simulink model "sm_car"  (R2024a)
settings: Solver=ode23t  StartTime=0.0  StopTime=25  MaxStep=0.4  RelTol=1e-3  AbsTol=1e-3  EnableMultiTasking=on
PreLoadFcn:
  | % Due to usability issue in Repeating Sequence block
  | warning('off','Simulink:Masking:Invalid');
  | 
  | % Eliminate unnecessary warnings in inactive variants
  | % Warnings generated only if you click through inactive variant
  | warning('off','MATLAB:nonExistentField');
  | warning('off','Simulink:Parameters:BlkParamUndefined');
PostLoadFcn:
  | set_param([bdroot '/Vehicle'],'popup_trailer','Off')
  | warning('off','sm:sli:setup:compile:LocalSolverNotSupported')
  | %sm_car_config_maneuver(bdroot,'WOT Braking');
  | sm_car_config_vehicle(bdroot,'false');
  | sm_car_config_logging(bdroot);
InitFcn:
  | sm_car_config_camera;
  | Vehicle = sm_car_vehcfg_checkConfig(Vehicle);
  | sm_car_check_tire_model(bdroot);
StartFcn:
  | tic;
StopFcn:
  | Elapsed_Sim_Time = toc;
  | % disp(['Elapsed Sim Time = ' num2str(Elapsed_Sim_Time)]);
values from neighbouring files (symbols this model uses):
  EFFECTIVE_ROLLING_RADIUS_OF_TIRES_M = 0.23323    [vehicle_specs.m]
  TARGET_SLIP_RATIO = 0.10    (= 0.1)    [vehicle_specs.m]
undefined symbols (not defined in the file or in its folder): Axle1D, AxleIn, Camera, Control, Driver, Init, Maneuver, MAXIMUM_CONTINUOUS_CURRENT_DRAW_A, MAXIMUM_NEGATIVE_TORQUE_FROM_MOTOR_Nm, MAXIMUM_TORQUE_FROM_MOTOR_Nm, Pedal, RaceFix, RaceSpin, Scene, ShaftL1, ShaftL2, ShaftR1, ShaftR2, Visual, X, xy_data_car_side, Y, Z
libraries: sm_lib x1112, nesl_utility x285, fl_lib x221, simulink x24, sdl_lib x16, SimscapeFluids_lib x9, ee_lib x5, Linkage_Systems x4, Tire_1x2x x4, simulink_extras x3, slpidlib x2, AntiRollBar_Systems x2
(part 9 of 43)

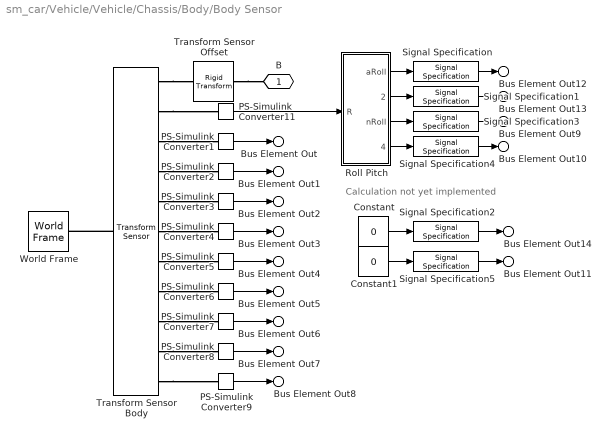
== system sm_car/Vehicle/Vehicle/Chassis/Body/Body Sensor ==
  note: Calculation not yet implemented
  Constant : Constant  Value=0
  Constant1 : Constant  Value=0
  PS-Simulink Converter1 : nesl_utility/PS-Simulink Converter  PhysicalDomain=network_engine_domain  SubClassName=ps_output  LeftPortType=input  RightPortType=output  PseudoPeriodic=off  Frequencies=[]  VectorFormat=1-D array  Unit=m  AffineConversion=off
  PS-Simulink Converter11 : nesl_utility/PS-Simulink Converter  PhysicalDomain=network_engine_domain  SubClassName=ps_output  LeftPortType=input  RightPortType=output  PseudoPeriodic=off  Frequencies=[]  VectorFormat=1-D array  Unit=1  AffineConversion=off
  PS-Simulink Converter2 : nesl_utility/PS-Simulink Converter  PhysicalDomain=network_engine_domain  SubClassName=ps_output  LeftPortType=input  RightPortType=output  PseudoPeriodic=off  Frequencies=[]  VectorFormat=1-D array  Unit=m  AffineConversion=off
  PS-Simulink Converter3 : nesl_utility/PS-Simulink Converter  PhysicalDomain=network_engine_domain  SubClassName=ps_output  LeftPortType=input  RightPortType=output  PseudoPeriodic=off  Frequencies=[]  VectorFormat=1-D array  Unit=m  AffineConversion=off
  PS-Simulink Converter4 : nesl_utility/PS-Simulink Converter  PhysicalDomain=network_engine_domain  SubClassName=ps_output  LeftPortType=input  RightPortType=output  PseudoPeriodic=off  Frequencies=[]  VectorFormat=1-D array  Unit=m/s  AffineConversion=off
  PS-Simulink Converter5 : nesl_utility/PS-Simulink Converter  PhysicalDomain=network_engine_domain  SubClassName=ps_output  LeftPortType=input  RightPortType=output  PseudoPeriodic=off  Frequencies=[]  VectorFormat=1-D array  Unit=m/s  AffineConversion=off
  PS-Simulink Converter6 : nesl_utility/PS-Simulink Converter  PhysicalDomain=network_engine_domain  SubClassName=ps_output  LeftPortType=input  RightPortType=output  PseudoPeriodic=off  Frequencies=[]  VectorFormat=1-D array  Unit=m/s  AffineConversion=off
  PS-Simulink Converter7 : nesl_utility/PS-Simulink Converter  PhysicalDomain=network_engine_domain  SubClassName=ps_output  LeftPortType=input  RightPortType=output  PseudoPeriodic=off  Frequencies=[]  VectorFormat=1-D array  Unit=m/s^2  AffineConversion=off
  PS-Simulink Converter8 : nesl_utility/PS-Simulink Converter  PhysicalDomain=network_engine_domain  SubClassName=ps_output  LeftPortType=input  RightPortType=output  PseudoPeriodic=off  Frequencies=[]  VectorFormat=1-D array  Unit=m/s^2  AffineConversion=off
  PS-Simulink Converter9 : nesl_utility/PS-Simulink Converter  PhysicalDomain=network_engine_domain  SubClassName=ps_output  LeftPortType=input  RightPortType=output  PseudoPeriodic=off  Frequencies=[]  VectorFormat=1-D array  Unit=m/s^2  AffineConversion=off
  Roll Pitch : Subsystem
  Signal Specification : SignalSpecification  Unit=rad
  Signal Specification1 : SignalSpecification  Unit=rad
  Signal Specification2 : SignalSpecification  Unit=rad
  Signal Specification3 : SignalSpecification  Unit=rad/s
  Signal Specification4 : SignalSpecification  Unit=rad/s
  Signal Specification5 : SignalSpecification  Unit=rad/s
  Transform Sensor Offset : sm_lib/Frames and Transforms/Rigid Transform  RotationMethod=None  FollAlignAxisA=+X  BaseAlignAxisA=+Y  FollAlignAxisB=+Y  BaseAlignAxisB=+Z  RotationStandardAxis=+Z  RotationAngle=0.0  RotationAngleUnits=deg  RotationArbitraryAxis=[0 0 1]  RotationSequenceAxes=FollowerAxes  RotationSequence=XYX  RotationSequenceAngles=[0 0 0]  RotationSequenceAnglesUnits=deg  RotationMatrix=[1 0 0; 0 1 0; 0 0 1]  Quaternion=[1 0 0 0]  TranslationMethod=Cartesian  TranslationCartesianOffset=offset_body_sensor  TranslationCartesianOffsetUnits=m  TranslationStandardAxis=+Z  TranslationStandardOffset=0  TranslationStandardOffsetUnits=m  TranslationROffset=0  TranslationROffsetUnits=m  TranslationThetaOffset=0  TranslationThetaOffsetUnits=deg  TranslationZOffset=0  TranslationZOffsetUnits=m
  Transform Sensor Body : sm_lib/Frames and Transforms/Transform Sensor  MeasurementFrame=NonRotatingFollower  RotationSequence=XYX  SenseAngle=off  SenseAxis=off  SenseQ=off  SenseR=on  SenseRotationSequence=off  SenseOmegaX=off  SenseOmegaY=off  SenseOmegaZ=off  SenseOmega=off  SenseQDot=off  SenseRDot=off  SenseRotationSequenceDot=off  SenseAlphaX=off  SenseAlphaY=off  SenseAlphaZ=off  SenseAlpha=off  SenseQDDot=off  SenseRDDot=off  SenseX=on  SenseY=on  SenseZ=on  SenseXYZ=off  SenseRad=off  SenseAzim=off  SenseDist=off  SenseInc=off  SenseXDot=on  SenseYDot=on  SenseZDot=on  SenseXYZDot=off  SenseRadDot=off  SenseAzimDot=off  SenseDistDot=off  SenseIncDot=off  SenseXDDot=on  SenseYDDot=on  SenseZDDot=on  SenseXYZDDot=off  SenseRadDDot=off  SenseAzimDDot=off  SenseDistDDot=off  SenseIncDDot=off
  World Frame : sm_lib/Frames and Transforms/World Frame
  B : PMIOPort  Side=Left
  Bus Element Out : Outport  VectorParamsAs1DForOutWhenUnconnected=off  PortName=Body  Element=x
  Bus Element Out1 : Outport  VectorParamsAs1DForOutWhenUnconnected=off  PortName=Body  Element=y
  Bus Element Out2 : Outport  VectorParamsAs1DForOutWhenUnconnected=off  PortName=Body  Element=z
  Bus Element Out3 : Outport  VectorParamsAs1DForOutWhenUnconnected=off  PortName=Body  Element=vx
  Bus Element Out4 : Outport  VectorParamsAs1DForOutWhenUnconnected=off  PortName=Body  Element=vy
  Bus Element Out5 : Outport  VectorParamsAs1DForOutWhenUnconnected=off  PortName=Body  Element=vz
  Bus Element Out6 : Outport  VectorParamsAs1DForOutWhenUnconnected=off  PortName=Body  Element=gx
  Bus Element Out7 : Outport  VectorParamsAs1DForOutWhenUnconnected=off  PortName=Body  Element=gy
  Bus Element Out8 : Outport  VectorParamsAs1DForOutWhenUnconnected=off  PortName=Body  Element=gz
  Bus Element Out9 : Outport  VectorParamsAs1DForOutWhenUnconnected=off  PortName=Body  Element=nRoll
  Bus Element Out10 : Outport  VectorParamsAs1DForOutWhenUnconnected=off  PortName=Body  Element=nPitch
  Bus Element Out11 : Outport  VectorParamsAs1DForOutWhenUnconnected=off  PortName=Body  Element=nYaw
  Bus Element Out12 : Outport  VectorParamsAs1DForOutWhenUnconnected=off  PortName=Body  Element=aRoll
  Bus Element Out13 : Outport  VectorParamsAs1DForOutWhenUnconnected=off  PortName=Body  Element=aPitch
  Bus Element Out14 : Outport  VectorParamsAs1DForOutWhenUnconnected=off  PortName=Body  Element=aYaw
  wires:
  PS-Simulink Converter9/1 -> Bus Element Out8/1
  PS-Simulink Converter11/1 -> Roll Pitch/1(R)
  PS-Simulink Converter6/1 -> Bus Element Out5/1
  PS-Simulink Converter7/1 -> Bus Element Out6/1
  PS-Simulink Converter2/1 -> Bus Element Out1/1
  PS-Simulink Converter8/1 -> Bus Element Out7/1
  PS-Simulink Converter5/1 -> Bus Element Out4/1
  PS-Simulink Converter3/1 -> Bus Element Out2/1
  PS-Simulink Converter1/1 -> Bus Element Out/1
  PS-Simulink Converter4/1 -> Bus Element Out3/1
  Signal Specification/1 -> Bus Element Out12/1
  Signal Specification1/1 -> Bus Element Out13/1
  Signal Specification2/1 -> Bus Element Out14/1
  Signal Specification3/1 -> Bus Element Out9/1
  Signal Specification4/1 -> Bus Element Out10/1
  Signal Specification5/1 -> Bus Element Out11/1
  Constant/1 -> Signal Specification2/1
  Constant1/1 -> Signal Specification5/1
  Roll Pitch/3(nRoll) -> Signal Specification3/1
  Roll Pitch/4(nPitch) -> Signal Specification4/1
  Roll Pitch/2(aPitch) -> Signal Specification1/1
  Roll Pitch/1(aRoll) -> Signal Specification/1
  connections:
  Transform Sensor Body/RConn5 -- PS-Simulink Converter3/LConn1
  Transform Sensor Body/RConn4 -- PS-Simulink Converter2/LConn1
  Transform Sensor Body/RConn11 -- PS-Simulink Converter9/LConn1
  Transform Sensor Body/RConn2 -- PS-Simulink Converter11/LConn1
  Transform Sensor Body/RConn7 -- PS-Simulink Converter5/LConn1
  Transform Sensor Body/RConn3 -- PS-Simulink Converter1/LConn1
  Transform Sensor Body/LConn1 -- World Frame/RConn1
  Transform Sensor Offset/LConn1 -- B/RConn1
  Transform Sensor Body/RConn10 -- PS-Simulink Converter8/LConn1
  Transform Sensor Body/RConn9 -- PS-Simulink Converter7/LConn1
  Transform Sensor Body/RConn8 -- PS-Simulink Converter6/LConn1
  Transform Sensor Body/RConn6 -- PS-Simulink Converter4/LConn1
  Transform Sensor Body/RConn1 -- Transform Sensor Offset/RConn1

== system sm_car/Vehicle/Vehicle/Chassis/Body/Passenger FL ==
  None : Subsystem  VariantControl=None
      mask Display: disp(' ')
  P : PMIOPort  Side=Left
  m : Outport  VectorParamsAs1DForOutWhenUnconnected=off

== system sm_car/Vehicle/Vehicle/Chassis/Body/Passenger FR ==
  None : Subsystem  VariantControl=None
      mask Display: disp(' ')
  P : PMIOPort  Side=Left
  m : Outport  VectorParamsAs1DForOutWhenUnconnected=off

== system sm_car/Vehicle/Vehicle/Chassis/Body/Passenger RL ==
  None : Subsystem  VariantControl=None
      mask Display: disp(' ')
  P : PMIOPort  Side=Left
  m : Outport  VectorParamsAs1DForOutWhenUnconnected=off

== system sm_car/Vehicle/Vehicle/Chassis/Body/Passenger RR ==
  None : Subsystem  VariantControl=None
      mask Display: disp(' ')
  P : PMIOPort  Side=Left
  m : Outport  VectorParamsAs1DForOutWhenUnconnected=off

== system sm_car/Vehicle/Vehicle/Chassis/Damper/Decoupled ==
  In Bus Element1 : Inport  PortName=Ctrl  Element=L1
  In Bus Element : Inport  PortName=Ctrl  Element=R1
  In Bus Element2 : Inport  PortName=Ctrl  Element=L2
  In Bus Element3 : Inport  PortName=Ctrl  Element=R2
  Damper A1 Heave : Subsystem  Variant=on  VariantControlMode=label  VariantControl=Variant1  LabelModeActiveChoice=Linear  mask(Variants for Damper){Damper=Damper.Axle1.Heave, VariantLabel=Damper.Axle1.Heave.class.Value}
      mask prompts: Damper "Damper Parameters"; VariantLabel "Variant Label"
      mask help: Select option and provide parameters for damper. Option is chosen by string provided in Variant Label. The parameters for the selected option is contained in Damper data structure.
      mask init:
      | curblk = gcb;
      | 
      | % Set variant for this block 
      | set_param(curblk,'LabelModeActiveChoice',VariantLabel);
      settings: AttributesFormatString=%<ActiveVariant>
      mask Display: disp(' ')
  Damper A1 Roll : Subsystem  Variant=on  VariantControlMode=label  VariantControl=Variant1  LabelModeActiveChoice=Linear  mask(Variants for Damper){Damper=Damper.Axle1.Roll, VariantLabel=Damper.Axle1.Roll.class.Value}
      mask prompts: Damper "Damper Parameters"; VariantLabel "Variant Label"
      mask help: Select option and provide parameters for damper. Option is chosen by string provided in Variant Label. The parameters for the selected option is contained in Damper data structure.
      mask init:
      | curblk = gcb;
      | 
      | % Set variant for this block 
      | set_param(curblk,'LabelModeActiveChoice',VariantLabel);
      settings: AttributesFormatString=%<ActiveVariant>
      mask Display: disp(' ')
  Damper A2 Heave : Subsystem  Variant=on  VariantControlMode=label  VariantControl=Variant1  LabelModeActiveChoice=Linear  mask(Variants for Damper){Damper=Damper.Axle2.Heave, VariantLabel=Damper.Axle2.Heave.class.Value}
      mask prompts: Damper "Damper Parameters"; VariantLabel "Variant Label"
      mask help: Select option and provide parameters for damper. Option is chosen by string provided in Variant Label. The parameters for the selected option is contained in Damper data structure.
      mask init:
      | curblk = gcb;
      | 
      | % Set variant for this block 
      | set_param(curblk,'LabelModeActiveChoice',VariantLabel);
      settings: AttributesFormatString=%<ActiveVariant>
      mask Display: disp(' ')
  Damper A2 Roll : Subsystem  Variant=on  VariantControlMode=label  VariantControl=Variant1  LabelModeActiveChoice=Linear  mask(Variants for Damper){Damper=Damper.Axle2.Roll, VariantLabel=Damper.Axle2.Roll.class.Value}
      mask prompts: Damper "Damper Parameters"; VariantLabel "Variant Label"
      mask help: Select option and provide parameters for damper. Option is chosen by string provided in Variant Label. The parameters for the selected option is contained in Damper data structure.
      mask init:
      | curblk = gcb;
      | 
      | % Set variant for this block 
      | set_param(curblk,'LabelModeActiveChoice',VariantLabel);
      settings: AttributesFormatString=%<ActiveVariant>
      mask Display: disp(' ')
  MTRef L1 : fl_lib/Mechanical/Translational Elements/Mechanical Translational Reference
  MTRef L2 : fl_lib/Mechanical/Translational Elements/Mechanical Translational Reference
  MTRef R1 : fl_lib/Mechanical/Translational Elements/Mechanical Translational Reference
  MTRef R2 : fl_lib/Mechanical/Translational Elements/Mechanical Translational Reference
  L1 : PMIOPort  Side=Left
  R1 : PMIOPort  Port=2  Side=Right
  L2 : PMIOPort  Port=3  Side=Left
  R2 : PMIOPort  Port=4  Side=Right
  Out Bus Element : Outport  VectorParamsAs1DForOutWhenUnconnected=off  PortName=meas  Element=L1
  Out Bus Element1 : Outport  VectorParamsAs1DForOutWhenUnconnected=off  PortName=meas  Element=R1
  Out Bus Element2 : Outport  VectorParamsAs1DForOutWhenUnconnected=off  PortName=meas  Element=L2
  Out Bus Element3 : Outport  VectorParamsAs1DForOutWhenUnconnected=off  PortName=meas  Element=R2
  wires:
  In Bus Element/1 -> Damper A1 Roll/1("Ctrl ")
  In Bus Element1/1 -> Damper A1 Heave/1("Ctrl ")
  Damper A1 Heave/1(" meas") -> Out Bus Element/1
  Damper A1 Roll/1(" meas") -> Out Bus Element1/1
  In Bus Element3/1 -> Damper A2 Roll/1("Ctrl ")
  In Bus Element2/1 -> Damper A2 Heave/1("Ctrl ")
  Damper A2 Heave/1(" meas") -> Out Bus Element2/1
  Damper A2 Roll/1(" meas") -> Out Bus Element3/1
  connections:
  Damper A1 Roll/LConn1 -- R1/RConn1
  Damper A1 Roll/RConn1 -- MTRef R1/LConn1
  Damper A2 Roll/LConn1 -- R2/RConn1
  Damper A2 Roll/RConn1 -- MTRef R2/LConn1
  Damper A2 Heave/LConn1 -- L2/RConn1
  Damper A2 Heave/RConn1 -- MTRef L2/LConn1
  Damper A1 Heave/LConn1 -- L1/RConn1
  Damper A1 Heave/RConn1 -- MTRef L1/LConn1

== system sm_car/Vehicle/Vehicle/Chassis/Damper/Independent ==
  In Bus Element1 : Inport  PortName=Ctrl  Element=L1
  In Bus Element : Inport  PortName=Ctrl  Element=R1
  In Bus Element2 : Inport  PortName=Ctrl  Element=L2
  In Bus Element3 : Inport  PortName=Ctrl  Element=R2
  Damper L1 : Subsystem  Variant=on  VariantControlMode=label  VariantControl=Variant1  LabelModeActiveChoice=Linear  mask(Variants for Damper){Damper=Damper.Axle1, VariantLabel=Damper.Axle1.class.Value}
      mask prompts: Damper "Damper Parameters"; VariantLabel "Variant Label"
      mask help: Select option and provide parameters for damper. Option is chosen by string provided in Variant Label. The parameters for the selected option is contained in Damper data structure.
      mask init:
      | curblk = gcb;
      | 
      | % Set variant for this block 
      | set_param(curblk,'LabelModeActiveChoice',VariantLabel);
      settings: AttributesFormatString=%<ActiveVariant>
      mask Display: disp(' ')
  Damper L2 : Subsystem  Variant=on  VariantControlMode=label  VariantControl=Variant1  LabelModeActiveChoice=Linear  mask(Variants for Damper){Damper=Damper.Axle2, VariantLabel=Damper.Axle2.class.Value}
      mask prompts: Damper "Damper Parameters"; VariantLabel "Variant Label"
      mask help: Select option and provide parameters for damper. Option is chosen by string provided in Variant Label. The parameters for the selected option is contained in Damper data structure.
      mask init:
      | curblk = gcb;
      | 
      | % Set variant for this block 
      | set_param(curblk,'LabelModeActiveChoice',VariantLabel);
      settings: AttributesFormatString=%<ActiveVariant>
      mask Display: disp(' ')
  Damper R1 : Subsystem  Variant=on  VariantControlMode=label  VariantControl=Variant1  LabelModeActiveChoice=Linear  mask(Variants for Damper){Damper=Damper.Axle1, VariantLabel=Damper.Axle1.class.Value}
      mask prompts: Damper "Damper Parameters"; VariantLabel "Variant Label"
      mask help: Select option and provide parameters for damper. Option is chosen by string provided in Variant Label. The parameters for the selected option is contained in Damper data structure.
      mask init:
      | curblk = gcb;
      | 
      | % Set variant for this block 
      | set_param(curblk,'LabelModeActiveChoice',VariantLabel);
      settings: AttributesFormatString=%<ActiveVariant>
      mask Display: disp(' ')
  Damper R2 : Subsystem  Variant=on  VariantControlMode=label  VariantControl=Variant1  LabelModeActiveChoice=Linear  mask(Variants for Damper){Damper=Damper.Axle2, VariantLabel=Damper.Axle2.class.Value}
      mask prompts: Damper "Damper Parameters"; VariantLabel "Variant Label"
      mask help: Select option and provide parameters for damper. Option is chosen by string provided in Variant Label. The parameters for the selected option is contained in Damper data structure.
      mask init:
      | curblk = gcb;
      | 
      | % Set variant for this block 
      | set_param(curblk,'LabelModeActiveChoice',VariantLabel);
      settings: AttributesFormatString=%<ActiveVariant>
      mask Display: disp(' ')
  MTRef L1 : fl_lib/Mechanical/Translational Elements/Mechanical Translational Reference
  MTRef L2 : fl_lib/Mechanical/Translational Elements/Mechanical Translational Reference
  MTRef R1 : fl_lib/Mechanical/Translational Elements/Mechanical Translational Reference
  MTRef R2 : fl_lib/Mechanical/Translational Elements/Mechanical Translational Reference
  L1 : PMIOPort  Side=Left
  R1 : PMIOPort  Port=2  Side=Right
  L2 : PMIOPort  Port=3  Side=Left
  R2 : PMIOPort  Port=4  Side=Right
  Out Bus Element : Outport  VectorParamsAs1DForOutWhenUnconnected=off  PortName=meas  Element=L1
  Out Bus Element1 : Outport  VectorParamsAs1DForOutWhenUnconnected=off  PortName=meas  Element=R1
  Out Bus Element2 : Outport  VectorParamsAs1DForOutWhenUnconnected=off  PortName=meas  Element=L2
  Out Bus Element3 : Outport  VectorParamsAs1DForOutWhenUnconnected=off  PortName=meas  Element=R2
  wires:
  In Bus Element/1 -> Damper R1/1("Ctrl ")
  In Bus Element1/1 -> Damper L1/1("Ctrl ")
  Damper L1/1(" meas") -> Out Bus Element/1
  Damper R1/1(" meas") -> Out Bus Element1/1
  In Bus Element3/1 -> Damper R2/1("Ctrl ")
  In Bus Element2/1 -> Damper L2/1("Ctrl ")
  Damper L2/1(" meas") -> Out Bus Element2/1
  Damper R2/1(" meas") -> Out Bus Element3/1
  connections:
  Damper R1/LConn1 -- R1/RConn1
  Damper R1/RConn1 -- MTRef R1/LConn1
  Damper R2/LConn1 -- R2/RConn1
  Damper R2/RConn1 -- MTRef R2/LConn1
  Damper L2/LConn1 -- L2/RConn1
  Damper L2/RConn1 -- MTRef L2/LConn1
  Damper L1/LConn1 -- L1/RConn1
  Damper L1/RConn1 -- MTRef L1/LConn1

== system sm_car/Vehicle/Vehicle/Chassis/Spring/Decoupled ==
  In Bus Element1 : Inport  PortName=Ctrl  Element=L1
  In Bus Element2 : Inport  PortName=Ctrl  Element=R1
  In Bus Element3 : Inport  PortName=Ctrl  Element=L2
  In Bus Element4 : Inport  PortName=Ctrl  Element=R2
  MTRef Heave A1 : fl_lib/Mechanical/Translational Elements/Mechanical Translational Reference
  MTRef Heave A2 : fl_lib/Mechanical/Translational Elements/Mechanical Translational Reference
  MTRef Roll A1 : fl_lib/Mechanical/Translational Elements/Mechanical Translational Reference
  MTRef Roll A2 : fl_lib/Mechanical/Translational Elements/Mechanical Translational Reference
  Spring A1 Heave : Subsystem  Variant=on  VariantControlMode=label  VariantControl=Variant1  LabelModeActiveChoice=Linear  mask(Variants for Spring){Spring=Spring.Axle1.Heave, VariantLabel=Spring.Axle1.Heave.class.Value}
      mask prompts: Spring "Spring Parameters"; VariantLabel "Variant Label"
      mask help: Select option and provide parameters for spring. Option is chosen by string provided in Variant Label. The parameters for the selected option is contained in Spring data structure.
      mask init:
      | curblk = gcb;
      | 
      | % Set variant for this block 
      | set_param(curblk,'LabelModeActiveChoice',VariantLabel);
      settings: AttributesFormatString=%<ActiveVariant>
      mask Display: disp(' ')
  Spring A1 Roll : Subsystem  Variant=on  VariantControlMode=label  VariantControl=Variant1  LabelModeActiveChoice=Linear  mask(Variants for Spring){Spring=Spring.Axle1.Roll, VariantLabel=Spring.Axle1.Roll.class.Value}
      mask prompts: Spring "Spring Parameters"; VariantLabel "Variant Label"
      mask help: Select option and provide parameters for spring. Option is chosen by string provided in Variant Label. The parameters for the selected option is contained in Spring data structure.
      mask init:
      | curblk = gcb;
      | 
      | % Set variant for this block 
      | set_param(curblk,'LabelModeActiveChoice',VariantLabel);
      settings: AttributesFormatString=%<ActiveVariant>
      mask Display: disp(' ')
  Spring A2 Heave : Subsystem  Variant=on  VariantControlMode=label  VariantControl=Variant1  LabelModeActiveChoice=Linear  mask(Variants for Spring){Spring=Spring.Axle2.Heave, VariantLabel=Spring.Axle2.Heave.class.Value}
      mask prompts: Spring "Spring Parameters"; VariantLabel "Variant Label"
      mask help: Select option and provide parameters for spring. Option is chosen by string provided in Variant Label. The parameters for the selected option is contained in Spring data structure.
      mask init:
      | curblk = gcb;
      | 
      | % Set variant for this block 
      | set_param(curblk,'LabelModeActiveChoice',VariantLabel);
      settings: AttributesFormatString=%<ActiveVariant>
      mask Display: disp(' ')
  Spring A2 Roll : Subsystem  Variant=on  VariantControlMode=label  VariantControl=Variant1  LabelModeActiveChoice=Linear  mask(Variants for Spring){Spring=Spring.Axle2.Roll, VariantLabel=Spring.Axle2.Roll.class.Value}
      mask prompts: Spring "Spring Parameters"; VariantLabel "Variant Label"
      mask help: Select option and provide parameters for spring. Option is chosen by string provided in Variant Label. The parameters for the selected option is contained in Spring data structure.
      mask init:
      | curblk = gcb;
      | 
      | % Set variant for this block 
      | set_param(curblk,'LabelModeActiveChoice',VariantLabel);
      settings: AttributesFormatString=%<ActiveVariant>
      mask Display: disp(' ')
  L1 : PMIOPort  Side=Left
  R1 : PMIOPort  Port=2  Side=Right
  L2 : PMIOPort  Port=3  Side=Left
  R2 : PMIOPort  Port=4  Side=Right
  Out Bus Element : Outport  VectorParamsAs1DForOutWhenUnconnected=off  PortName=meas  Element=L1
  Out Bus Element1 : Outport  VectorParamsAs1DForOutWhenUnconnected=off  PortName=meas  Element=R1
  Out Bus Element2 : Outport  VectorParamsAs1DForOutWhenUnconnected=off  PortName=meas  Element=L2
  Out Bus Element3 : Outport  VectorParamsAs1DForOutWhenUnconnected=off  PortName=meas  Element=R2
  wires:
  In Bus Element1/1 -> Spring A1 Heave/1("Ctrl ")
  Spring A1 Heave/1(" meas") -> Out Bus Element/1
  In Bus Element2/1 -> Spring A1 Roll/1("Ctrl ")
  Spring A1 Roll/1(" meas") -> Out Bus Element1/1
  In Bus Element3/1 -> Spring A2 Heave/1("Ctrl ")
  Spring A2 Heave/1(" meas") -> Out Bus Element2/1
  In Bus Element4/1 -> Spring A2 Roll/1("Ctrl ")
  Spring A2 Roll/1(" meas") -> Out Bus Element3/1
  connections:
  Spring A1 Roll/LConn1 -- R1/RConn1
  Spring A1 Roll/RConn1 -- MTRef Roll A1/LConn1
  Spring A2 Roll/LConn1 -- R2/RConn1
  Spring A2 Roll/RConn1 -- MTRef Roll A2/LConn1
  Spring A2 Heave/LConn1 -- L2/RConn1
  Spring A2 Heave/RConn1 -- MTRef Heave A2/LConn1
  Spring A1 Heave/LConn1 -- L1/RConn1
  Spring A1 Heave/RConn1 -- MTRef Heave A1/LConn1

== system sm_car/Vehicle/Vehicle/Chassis/Spring/Independent ==
  In Bus Element1 : Inport  PortName=Ctrl  Element=L1
  In Bus Element2 : Inport  PortName=Ctrl  Element=R1
  In Bus Element3 : Inport  PortName=Ctrl  Element=L2
  In Bus Element4 : Inport  PortName=Ctrl  Element=R2
  MTRef L1 : fl_lib/Mechanical/Translational Elements/Mechanical Translational Reference
  MTRef L2 : fl_lib/Mechanical/Translational Elements/Mechanical Translational Reference
  MTRef R1 : fl_lib/Mechanical/Translational Elements/Mechanical Translational Reference
  MTRef R2 : fl_lib/Mechanical/Translational Elements/Mechanical Translational Reference
  Spring L1 : Subsystem  Variant=on  VariantControlMode=label  VariantControl=Variant1  LabelModeActiveChoice=Linear  mask(Variants for Spring){Spring=Spring.Axle1, VariantLabel=Spring.Axle1.class.Value}
      mask prompts: Spring "Spring Parameters"; VariantLabel "Variant Label"
      mask help: Select option and provide parameters for spring. Option is chosen by string provided in Variant Label. The parameters for the selected option is contained in Spring data structure.
      mask init:
      | curblk = gcb;
      | 
      | % Set variant for this block 
      | set_param(curblk,'LabelModeActiveChoice',VariantLabel);
      settings: AttributesFormatString=%<ActiveVariant>
      mask Display: disp(' ')
  Spring L2 : Subsystem  Variant=on  VariantControlMode=label  VariantControl=Variant1  LabelModeActiveChoice=Linear  mask(Variants for Spring){Spring=Spring.Axle2, VariantLabel=Spring.Axle2.class.Value}
      mask prompts: Spring "Spring Parameters"; VariantLabel "Variant Label"
      mask help: Select option and provide parameters for spring. Option is chosen by string provided in Variant Label. The parameters for the selected option is contained in Spring data structure.
      mask init:
      | curblk = gcb;
      | 
      | % Set variant for this block 
      | set_param(curblk,'LabelModeActiveChoice',VariantLabel);
      settings: AttributesFormatString=%<ActiveVariant>
      mask Display: disp(' ')
  Spring R1 : Subsystem  Variant=on  VariantControlMode=label  VariantControl=Variant1  LabelModeActiveChoice=Linear  mask(Variants for Spring){Spring=Spring.Axle1, VariantLabel=Spring.Axle1.class.Value}
      mask prompts: Spring "Spring Parameters"; VariantLabel "Variant Label"
      mask help: Select option and provide parameters for spring. Option is chosen by string provided in Variant Label. The parameters for the selected option is contained in Spring data structure.
      mask init:
      | curblk = gcb;
      | 
      | % Set variant for this block 
      | set_param(curblk,'LabelModeActiveChoice',VariantLabel);
      settings: AttributesFormatString=%<ActiveVariant>
      mask Display: disp(' ')
  Spring R2 : Subsystem  Variant=on  VariantControlMode=label  VariantControl=Variant1  LabelModeActiveChoice=Linear  mask(Variants for Spring){Spring=Spring.Axle2, VariantLabel=Spring.Axle2.class.Value}
      mask prompts: Spring "Spring Parameters"; VariantLabel "Variant Label"
      mask help: Select option and provide parameters for spring. Option is chosen by string provided in Variant Label. The parameters for the selected option is contained in Spring data structure.
      mask init:
      | curblk = gcb;
      | 
      | % Set variant for this block 
      | set_param(curblk,'LabelModeActiveChoice',VariantLabel);
      settings: AttributesFormatString=%<ActiveVariant>
      mask Display: disp(' ')
  L1 : PMIOPort  Side=Left
  R1 : PMIOPort  Port=2  Side=Right
  L2 : PMIOPort  Port=3  Side=Left
  R2 : PMIOPort  Port=4  Side=Right
  Out Bus Element : Outport  VectorParamsAs1DForOutWhenUnconnected=off  PortName=meas  Element=L1
  Out Bus Element1 : Outport  VectorParamsAs1DForOutWhenUnconnected=off  PortName=meas  Element=R1
  Out Bus Element2 : Outport  VectorParamsAs1DForOutWhenUnconnected=off  PortName=meas  Element=L2
  Out Bus Element3 : Outport  VectorParamsAs1DForOutWhenUnconnected=off  PortName=meas  Element=R2
  wires:
  In Bus Element1/1 -> Spring L1/1("Ctrl ")
  Spring L1/1(" meas") -> Out Bus Element/1
  In Bus Element2/1 -> Spring R1/1("Ctrl ")
  Spring R1/1(" meas") -> Out Bus Element1/1
  In Bus Element3/1 -> Spring L2/1("Ctrl ")
  Spring L2/1(" meas") -> Out Bus Element2/1
  In Bus Element4/1 -> Spring R2/1("Ctrl ")
  Spring R2/1(" meas") -> Out Bus Element3/1
  connections:
  Spring R1/LConn1 -- R1/RConn1
  Spring R1/RConn1 -- MTRef R1/LConn1
  Spring R2/LConn1 -- R2/RConn1
  Spring R2/RConn1 -- MTRef R2/LConn1
  Spring L2/LConn1 -- L2/RConn1
  Spring L2/RConn1 -- MTRef L2/LConn1
  Spring L1/LConn1 -- L1/RConn1
  Spring L1/RConn1 -- MTRef L1/LConn1

== system sm_car/Vehicle/Vehicle/Chassis/SuspA1/Linkage ==
  In Bus Element : Inport  PortName=CtrlBus  Element=Steer
  DrvBus : Inport  Port=2
  Anti Roll Bar : AntiRollBar_Systems/Anti Roll Bar  LabelModeActiveChoice=Droplink  AntiRollBar=Susp.AntiRollBar  VariantLabel=Susp.AntiRollBar.class.Value
      settings: AttributesFormatString=%<LabelModeActiveChoice>
  Linkage L : Linkage_Systems/Linkage  VariantControl=Variant1  LabelModeActiveChoice=DoubleWishbone  popup_leftRight=Left  Linkage=Susp.Linkage  InitLinkage=Init  VariantLabel=Susp.Linkage.class.Value
      settings: AttributesFormatString=%<ActiveVariant>
  Linkage R : Linkage_Systems/Linkage  Tag=PublishSubsystem  VariantControl=Variant1  LabelModeActiveChoice=DoubleWishbone  popup_leftRight=Right  Linkage=Susp.Linkage  InitLinkage=Init  VariantLabel=Susp.Linkage.class.Value
      settings: AttributesFormatString=%<ActiveVariant>
  Simscape Bus L : SimscapeBus  HierarchyStrings=RaceSpin;RaceFix;Axle1D;AxleIn
  Simscape Bus L1 : SimscapeBus  HierarchyStrings=RaceSpin;RaceFix;Axle1D;AxleIn
  Steer : Subsystem  Variant=on  VariantControlMode=label  VariantControl=Steer  LabelModeActiveChoice=WheelDrivenRack1UJoint  mask{Steer=Susp.Steer, VariantLabel=Susp.Steer.class.Value}
      mask prompts: Steer "Steer Parameters"; VariantLabel "Variant Label"
      mask init:
      | curblk = gcb;
      | 
      | % Set variant for this block 
      | set_param(curblk,'LabelModeActiveChoice',VariantLabel);
      settings: AttributesFormatString=%<ActiveVariant>
      mask Display: disp(' ');
  Wheel Meas Left : Subsystem  mask(Wheel Measurements){popup_leftRight=Left}
      mask prompts: popup_leftRight "Left/Right"
      mask help: Calculates toe and camber angles based on orientation of wheel spin axis. To estimate steering axis inclination, the same measurements are done along the longitudinal axis (X) of the tire. Set Left/Right so that the sign of the logged toe and camber angles is associated with towards/away from vehicle center.
      mask init:
      | if(popup_leftRight == 1)
      |     rhs_tc = 1;
      | elseif(popup_leftRight == 2)
      |     rhs_tc = -1;
      | end
      mask TypeOptions popup_leftRight: Left | Right
  Wheel Meas Right : Subsystem  mask(Wheel Measurements){popup_leftRight=Right}
      mask prompts: popup_leftRight "Left/Right"
      mask help: Calculates toe and camber angles based on orientation of wheel spin axis. To estimate steering axis inclination, the same measurements are done along the longitudinal axis (X) of the tire. Set Left/Right so that the sign of the logged toe and camber angles is associated with towards/away from vehicle center.
      mask init:
      | if(popup_leftRight == 1)
      |     rhs_tc = 1;
      | elseif(popup_leftRight == 2)
      |     rhs_tc = -1;
      | end
      mask TypeOptions popup_leftRight: Left | Right
  WCL : PMIOPort  Side=Left
  Ref : PMIOPort  Port=2  Side=Right
  WCR : PMIOPort  Port=3  Side=Right
  AxleL : PMIOPort  Port=4  Side=Left
  AxleR : PMIOPort  Port=5  Side=Right
  SprL : PMIOPort  Port=6  Side=Left
  SprR : PMIOPort  Port=7  Side=Right
  DmpL : PMIOPort  Port=8  Side=Left
  DmpR : PMIOPort  Port=9  Side=Right
  Out Bus Element : Outport  VectorParamsAs1DForOutWhenUnconnected=off  PortName=OutBus  Element=Steer
  Out Bus Element1 : Outport  VectorParamsAs1DForOutWhenUnconnected=off  PortName=OutBus  Element=AntiRollBar
  Out Bus Element2 : Outport  VectorParamsAs1DForOutWhenUnconnected=off  PortName=OutBus  Element=WhlL
  Out Bus Element3 : Outport  VectorParamsAs1DForOutWhenUnconnected=off  PortName=OutBus  Element=WhlR
  Out Bus Element4 : Outport  VectorParamsAs1DForOutWhenUnconnected=off  PortName=OutBus  Element=LinkageR
  Out Bus Element5 : Outport  VectorParamsAs1DForOutWhenUnconnected=off  PortName=OutBus  Element=LinkageL
  wires:
  Linkage L/1 -> Out Bus Element5/1
  Linkage R/1 -> Out Bus Element4/1
  DrvBus/1 -> Steer/1(DrvBus)
  Steer/1(" meas") -> Out Bus Element/1
  In Bus Element/1 -> Steer/2(CtrlBus)
  Anti Roll Bar/1 -> Out Bus Element1/1
  Wheel Meas Left/1(meas) -> Out Bus Element2/1
  Wheel Meas Right/1(meas) -> Out Bus Element3/1
  connections:
  Steer/RConn3 -- Linkage R/RConn1
  Ref/RConn1 -- Anti Roll Bar/LConn2 -- Linkage R/RConn2 -- Wheel Meas Right/LConn1 -- Wheel Meas Left/LConn1 -- Steer/RConn2 -- Linkage L/RConn2
  Linkage L/LConn1 -- WCL/RConn1 -- Wheel Meas Left/LConn2
  Linkage R/LConn1 -- WCR/RConn1 -- Wheel Meas Right/LConn2
  Steer/RConn1 -- Linkage L/RConn1
  DmpL/RConn1 -- Linkage L/LConn7
  Simscape Bus L/LConn4 -- Linkage L/LConn5
  Simscape Bus L/LConn1 -- Linkage L/LConn2
  Linkage L/LConn3 -- Simscape Bus L/LConn2
  Linkage L/LConn4 -- Simscape Bus L/LConn3
  AxleL/RConn1 -- Simscape Bus L/RConn1
  DmpR/RConn1 -- Linkage R/LConn7
  SprR/RConn1 -- Linkage R/LConn6
  Simscape Bus L1/LConn1 -- Linkage R/LConn2
  Simscape Bus L1/LConn2 -- Linkage R/LConn3
  Simscape Bus L1/LConn3 -- Linkage R/LConn4
  Simscape Bus L1/RConn1 -- AxleR/RConn1
  SprL/RConn1 -- Linkage L/LConn6
  Simscape Bus L1/LConn4 -- Linkage R/LConn5
  Anti Roll Bar/LConn3 -- Linkage R/LConn8
  Anti Roll Bar/LConn1 -- Linkage L/LConn8

== system sm_car/Vehicle/Vehicle/Chassis/SuspA1/Linkage Decoupled ==
  In Bus Element : Inport  PortName=CtrlBus  Element=Steer
  DrvBus : Inport  Port=2
  Linkage L : Linkage_Decoupled/Linkage  VariantControl=Variant1  LabelModeActiveChoice=DWDecoupled  popup_leftRight=Left  Linkage=Susp.Linkage  InitLinkage=Init  VariantLabel=Susp.Linkage.class.Value
      settings: AttributesFormatString=%<ActiveVariant>
  Linkage R : Linkage_Decoupled/Linkage  VariantControl=Variant1  LabelModeActiveChoice=DWDecoupled  popup_leftRight=Right  Linkage=Susp.Linkage  InitLinkage=Init  VariantLabel=Susp.Linkage.class.Value
      settings: AttributesFormatString=%<ActiveVariant>
  RollHeave Decouple : Subsystem  VariantControl=Variant1  mask(Roll and Heave Spring Dampers){hp_pushrod=Susp.Linkage.Pushrod.sBellcrank.Value, hp_bcr_pivot=Susp.Linkage.Bellcrank.sPivot.Value, hp_bcr_shock_heaveL=Susp.Linkage.Shock.Heave.sLeft.Value, hp_bcr_shock_heaveR=Susp.Linkage.Shock.Heave.sRight.Value, hp_bcr_shock_rollL=Susp.Linkage.Shock.Roll.sLeft.Value, hp_bcr_shock_rollR=Susp.Linkage.Shock.Roll.sRight.Value, shock_pist_mass_heave=Susp.Linkage.Shock.Heave.mPiston.Value, shock_pist_mass_roll=Susp.Linkage.Shock.Roll.mPiston.Value, shock_cyl_mass_heave=Susp.Linkage.Shock.Heave.mCylinder.Value, shock_cyl_mass_roll=Susp.Linkage.Shock.Roll.mCylinder.Value, up_lim_bumpstop_heave=Susp.Linkage.Endstop.Heave.xMax.Value, up_lim_bumpstop_roll=Susp.Linkage.Endstop.Roll.xMax.Value, low_lim_bumpstop_heave=Susp.Linkage.Endstop.Heave.xMin.Value, low_lim_bumpstop_roll=Susp.Linkage.Endstop.Roll.xMin.Value, clr_conn_shock=Visual.hp.clr, opc_conn_shock=Visual.hp.opc, size_conn_shock=Visual.hp.rad, clr_shock_cyl=Visual.Shock.cyl.clr, opc_shock_cyl=Visual.part.opc, radius_shock_cyl=Visual.Shock.cyl.rad, clr_shock_piston=Visual.Shock.piston.clr, opc_shock_piston=Visual.part.opc, clr_shock_bumpstop=Visual.Shock.bumpstop.clr, opc_shock_bumpstop=Visual.part.opc, deadvol_len_shock_cyl=Visual.Shock.dead_length, piston_len_shock=Visual.Shock.piston.len, cyl_cap_len_shock=Visual.Shock.cap.len, bumpstop_len_shock=Visual.Shock.bumpstop.len}
      mask prompts: hp_pushrod "HP Pushrod Inner  [xyz] (m)"; hp_bcr_pivot "HP Bellcrank Pivot [xyz] (m)"; deadvol_len_shock_cyl "Dead Volume Height (m)"; piston_len_shock "Piston Length (m)"; cyl_cap_len_shock "Cylinder Cap Length (m)"; bumpstop_len_shock "Bumpstop Length (m)"
      mask help: Models springs and dampers in a suspension design that decouples stiffness and damping for body roll and heave.
      mask init:
      | % Code to mirror hardpoint about vehicle xz plane
      | % and the plane defined by the bellcrank pivot axis
      | % and the y axis of the vehicle
      | % Code not used so that points can be specified independently
      | % Left here as a reference.
      | %{
      |  
      | a1 = atan2(hp_pushrod(1)-hp_bcr_pivot(1)   ,hp_pushrod(3)-hp_bcr_pivot(3));
      | a2 = atan2(hp_bcr_shock_roll(1)-hp_bcr_pivot(1),hp_bcr_shock_roll(3)-hp_bcr_pivot(3));
      | d_roll2piv = norm(hp_bcr_shock_roll([1 3])-hp_bcr_pivot([1 3]));
      | d_roll_mirror_axis = d_roll2piv*cos(a2-a1);
      | mirr_dx = d_roll_mirror_axis*sin(a1);
      | mirr_dz = d_roll_mirror_axis*cos(a1);
      | hp_bcr_shock_roll_r = ...
      |     [hp_bcr_shock_roll(1)-2*mirr_dx -hp_bcr_shock_roll(2) hp_bcr_shock_roll(3)-2*mirr_dz]
      | %}
      mask TypeOptions shock_pist_mass_heave: Shock Heave/shock_pist_mass
      mask TypeOptions shock_pist_mass_roll: Shock Roll/shock_pist_mass
      mask TypeOptions shock_cyl_mass_heave: Shock Heave/shock_cyl_mass
      mask TypeOptions shock_cyl_mass_roll: Shock Roll/shock_cyl_mass
      mask TypeOptions up_lim_bumpstop_heave: Shock Heave/up_lim_bumpstop
      mask TypeOptions up_lim_bumpstop_roll: Shock Roll/up_lim_bumpstop
      mask TypeOptions low_lim_bumpstop_heave: Shock Heave/low_lim_bumpstop
      mask TypeOptions low_lim_bumpstop_roll: Shock Roll/low_lim_bumpstop
      mask TypeOptions clr_conn_shock: Shock Heave/clr_conn_shock | Shock Roll/clr_conn_shock
      mask TypeOptions opc_conn_shock: Shock Heave/opc_conn_shock | Shock Roll/opc_conn_shock
      mask TypeOptions size_conn_shock: Shock Heave/size_conn_shock | Shock Roll/size_conn_shock
      mask TypeOptions clr_shock_cyl: Shock Heave/clr_shock_cyl | Shock Roll/clr_shock_cyl
      mask TypeOptions opc_shock_cyl: Shock Heave/opc_shock_cyl | Shock Roll/opc_shock_cyl
      mask TypeOptions radius_shock_cyl: Shock Heave/radius_shock_cyl | Shock Roll/radius_shock_cyl
      mask TypeOptions clr_shock_piston: Shock Heave/clr_shock_piston | Shock Roll/clr_shock_piston
      mask TypeOptions opc_shock_piston: Shock Heave/opc_shock_piston | Shock Roll/opc_shock_piston
      mask TypeOptions clr_shock_bumpstop: Shock Heave/clr_shock_bumpstop | Shock Roll/clr_shock_bumpstop
      mask TypeOptions opc_shock_bumpstop: Shock Heave/opc_shock_bumpstop | Shock Roll/opc_shock_bumpstop
      mask TypeOptions deadvol_len_shock_cyl: Shock Heave/deadvol_len_shock_cyl | Shock Roll/deadvol_len_shock_cyl
      mask TypeOptions piston_len_shock: Shock Heave/piston_len_shock | Shock Roll/piston_len_shock
      mask TypeOptions cyl_cap_len_shock: Shock Heave/cyl_cap_len_shock | Shock Roll/cyl_cap_len_shock
      mask TypeOptions bumpstop_len_shock: Shock Heave/bumpstop_len_shock | Shock Roll/bumpstop_len_shock
      mask DialogControl cont_hp Prompt: Hardpoints
      mask DialogControl text_hp_left Prompt: Left
      mask DialogControl text_hp_right Prompt: Right
      mask DialogControl text_hp_heave Prompt: Heave [xyz] (m)
      mask DialogControl text_hp_roll Prompt: Roll [xyz] (m)
      mask DialogControl cont_shock Prompt: Shock
      mask DialogControl text_shock_parts_blank Prompt: Parts
      mask DialogControl text_shock_heave Prompt: Heave
      mask DialogControl text_shock_roll Prompt: Roll
      mask DialogControl text_shock_pistm Prompt: Piston Mass (kg)
      mask DialogControl text_shock_cylm Prompt: Cylinder Mass (kg)
      mask DialogControl text_shock_bumpstop_par Prompt: Bumpstop
      mask DialogControl text_bump_ul Prompt: Upper Limit (m)
      mask DialogControl text_bump_low Prompt: Lower Limit (m)
      mask DialogControl cont_vis_shock Prompt: Visualization
      mask DialogControl text_clr_shock Prompt: Color  [RGB]
      mask DialogControl text_opc_shock Prompt: Opac. (0-1)
      mask DialogControl text_size_shock Prompt: Size (m)
      mask DialogControl text_conn_shock Prompt: Connections
      mask DialogControl text_shock_shock Prompt: Cylinder
      mask DialogControl text_shock_piston Prompt: Piston
      mask DialogControl text_piston_radius Prompt: <cylinder radius>
      mask DialogControl text_shock_bumpstop Prompt: Bumpstop
      mask DialogControl text_bumpstop_radius Prompt: <cylinder radius>
      mask Display: image('sm_car_vehicle_linkage_rollHeaveDecouple_IMAGE.png');
  Simscape Bus L : SimscapeBus  HierarchyStrings=RaceSpin;RaceFix;Axle1D;AxleIn
  Simscape Bus L1 : SimscapeBus  HierarchyStrings=RaceSpin;RaceFix;Axle1D;AxleIn
  Steer : Subsystem  Variant=on  VariantControlMode=label  VariantControl=Steer  LabelModeActiveChoice=WheelDrivenRack1UJoint  mask{Steer=Susp.Steer, VariantLabel=Susp.Steer.class.Value}
      mask prompts: Steer "Steer Parameters"; VariantLabel "Variant Label"
      mask init:
      | curblk = gcb;
      | 
      | % Set variant for this block 
      | set_param(curblk,'LabelModeActiveChoice',VariantLabel);
      settings: AttributesFormatString=%<ActiveVariant>
      mask Display: disp(' ');
  Wheel Meas Left : Subsystem  mask(Wheel Measurements){popup_leftRight=Left}
      mask prompts: popup_leftRight "Left/Right"
      mask help: Calculates toe and camber angles based on orientation of wheel spin axis. To estimate steering axis inclination, the same measurements are done along the longitudinal axis (X) of the tire. Set Left/Right so that the sign of the logged toe and camber angles is associated with towards/away from vehicle center.
      mask init:
      | if(popup_leftRight == 1)
      |     rhs_tc = 1;
      | elseif(popup_leftRight == 2)
      |     rhs_tc = -1;
      | end
      mask TypeOptions popup_leftRight: Left | Right
  Wheel Meas Right : Subsystem  mask(Wheel Measurements){popup_leftRight=Right}
      mask prompts: popup_leftRight "Left/Right"
      mask help: Calculates toe and camber angles based on orientation of wheel spin axis. To estimate steering axis inclination, the same measurements are done along the longitudinal axis (X) of the tire. Set Left/Right so that the sign of the logged toe and camber angles is associated with towards/away from vehicle center.
      mask init:
      | if(popup_leftRight == 1)
      |     rhs_tc = 1;
      | elseif(popup_leftRight == 2)
      |     rhs_tc = -1;
      | end
      mask TypeOptions popup_leftRight: Left | Right
  WCL : PMIOPort  Side=Left
  Ref : PMIOPort  Port=2  Side=Right
  WCR : PMIOPort  Port=3  Side=Right
  AxleL : PMIOPort  Port=4  Side=Left
  AxleR : PMIOPort  Port=5  Side=Right
  SprL : PMIOPort  Port=6  Side=Left
  SprR : PMIOPort  Port=7  Side=Right
  DmpL : PMIOPort  Port=8  Side=Left
  DmpR : PMIOPort  Port=9  Side=Right
  Out Bus Element : Outport  VectorParamsAs1DForOutWhenUnconnected=off  PortName=OutBus  Element=Steer
  Out Bus Element1 : Outport  VectorParamsAs1DForOutWhenUnconnected=off  PortName=OutBus  Element=RollHeave
  Out Bus Element2 : Outport  VectorParamsAs1DForOutWhenUnconnected=off  PortName=OutBus  Element=WhlL
  Out Bus Element3 : Outport  VectorParamsAs1DForOutWhenUnconnected=off  PortName=OutBus  Element=WhlR
  Out Bus Element4 : Outport  VectorParamsAs1DForOutWhenUnconnected=off  PortName=OutBus  Element=LinkageR
  Out Bus Element5 : Outport  VectorParamsAs1DForOutWhenUnconnected=off  PortName=OutBus  Element=LinkageL
  wires:
  Linkage L/1 -> Out Bus Element5/1
  Linkage R/1 -> Out Bus Element4/1
  RollHeave Decouple/1(meas) -> Out Bus Element1/1
  DrvBus/1 -> Steer/1(DrvBus)
  Steer/1(" meas") -> Out Bus Element/1
  In Bus Element/1 -> Steer/2(CtrlBus)
  Wheel Meas Left/1(meas) -> Out Bus Element2/1
  Wheel Meas Right/1(meas) -> Out Bus Element3/1
  connections:
  SprR/RConn1 -- RollHeave Decouple/LConn5
  DmpR/RConn1 -- RollHeave Decouple/LConn6
  SprL/RConn1 -- RollHeave Decouple/LConn3
  DmpL/RConn1 -- RollHeave Decouple/LConn4
  RollHeave Decouple/LConn8 -- Linkage R/LConn6
  RollHeave Decouple/LConn7 -- Linkage R/LConn7
  RollHeave Decouple/LConn2 -- Linkage L/LConn7
  Steer/RConn3 -- Linkage R/RConn1
  Linkage L/RConn2 -- Ref/RConn1 -- Linkage R/RConn2 -- Wheel Meas Left/LConn1 -- Wheel Meas Right/LConn1 -- Steer/RConn2
  WCL/RConn1 -- Linkage L/LConn1 -- Wheel Meas Left/LConn2
  WCR/RConn1 -- Linkage R/LConn1 -- Wheel Meas Right/LConn2
  Steer/RConn1 -- Linkage L/RConn1
  Linkage L/LConn5 -- Simscape Bus L/LConn4
  Linkage L/LConn2 -- Simscape Bus L/LConn1
  Linkage L/LConn3 -- Simscape Bus L/LConn2
  Linkage L/LConn4 -- Simscape Bus L/LConn3
  AxleL/RConn1 -- Simscape Bus L/RConn1
  Linkage R/LConn2 -- Simscape Bus L1/LConn1
  Linkage R/LConn3 -- Simscape Bus L1/LConn2
  Linkage R/LConn4 -- Simscape Bus L1/LConn3
  Simscape Bus L1/RConn1 -- AxleR/RConn1
  Linkage R/LConn5 -- Simscape Bus L1/LConn4
  RollHeave Decouple/LConn1 -- Linkage L/LConn6
